simulink model "tp320031"  (Simulink 3.0)
settings: Solver=ode1  SolverMode=SingleTasking  StartTime=0.0  StopTime=t_sim  FixedStep=Ts  RelTol=1e-3
values from neighbouring files (symbols this model uses):
  t_prep = 80    [step_resp1.mat]
  Ts = 0.2    [init_I0_disc2.m]    (also in init_PI0_windupless.m = 0.5; init_PI1_windupless.m; init_PID.m; step_resp1.mat)
  Umax = 5    [init_I0_disc2.m]    (also in init_PI0_windupless.m; init_PI1_windupless.m; init_PID.m; step_resp1.mat)
  Umin = 0    [init_I0_disc2.m]    (also in init_PI0_windupless.m; init_PI1_windupless.m; init_PID.m; step_resp1.mat)
  w = 20    [step_resp1.mat]
undefined symbols (not defined in the file or in its folder): t_step
libraries: udaq28LT_lib x1
settings Model: LastModifiedBy=mato  SaveFormat=Matrix  BooleanDataType=on

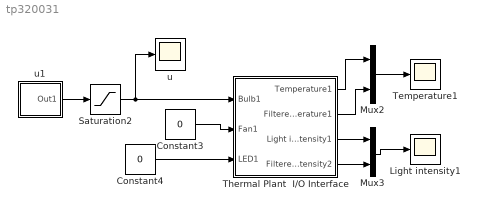
== system tp320031 ==
  Constant3 : Constant  Value=0
  Constant4 : Constant  Value=0
  Light intensity1 : Scope
      settings: TickLabels=on  TimeRange=30  YMin=0  YMax=100  SaveName=yl  DataFormat=Matrix
  Mux2 : Mux  Inputs=2
  Mux3 : Mux  Inputs=2
  Saturation2 : Saturate  UpperLimit=Umax  LowerLimit=Umin
  Temperature1 : Scope
      settings: TickLabels=on  TimeRange=30  YMin=15  YMax=50  SaveName=yt  DataFormat=Matrix
  Thermal Plant  I/O Interface : Subsystem
      mask Display: disp('Thermo-optical\nPlant\nI/O Interface')
  u : Scope
      settings: TimeRange=33  YMin=-0.5  YMax=5.5  SaveName=u  DataFormat=Matrix  Decimation=10  SampleInput=on  SampleTime=Ts
  u1 : Subsystem
  wires:
  Saturation2/1 -> u/1, Thermal Plant  I/O Interface/1(Bulb1)
  u1/1(Out1) -> Saturation2/1
  Mux3/1 -> Light intensity1/1
  Mux2/1 -> Temperature1/1
  Constant3/1 -> Thermal Plant  I/O Interface/2(Fan1)
  Constant4/1 -> Thermal Plant  I/O Interface/3(LED1)
  Thermal Plant  I/O Interface/1(Temperature1) -> Mux2/1
  Thermal Plant  I/O Interface/2(Filtered  temperature1) -> Mux2/2
  Thermal Plant  I/O Interface/3(Light intensity1) -> Mux3/1
  Thermal Plant  I/O Interface/4(Filtered  light intensity2) -> Mux3/2

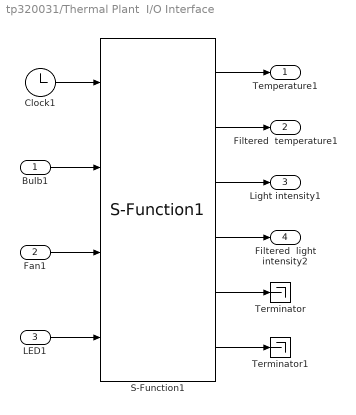
== system tp320031/Thermal Plant  I/O Interface ==
  Bulb1 : Inport  Port=1  PortWidth=-1  SampleTime=-1  DataType=auto
      settings: SignalType=auto
  Fan1 : Inport  Port=2  PortWidth=-1  SampleTime=-1  DataType=auto
      settings: SignalType=auto
  LED1 : Inport  Port=3  PortWidth=-1  SampleTime=-1  DataType=auto
      settings: SignalType=auto
  Clock1 : Clock
      settings: DisplayTime=off  Decimation=10
  S-Function1 : udaq28LT_lib/S-Function1  Priority=1  com_port=COM3  Ts=Ts  events_ot=2  rd_timeout=Ts/2*1000  matlab_prior=ABOVE_NORMAL_PRIORITY  warning=on  printout=off
  Terminator : Terminator
  Terminator1 : Terminator
  Temperature1 : Outport  Port=1
  Filtered  temperature1 : Outport  Port=2
  Light intensity1 : Outport  Port=3
  Filtered  light intensity2 : Outport  Port=4
  wires:
  S-Function1/1 -> Temperature1/1
  S-Function1/2 -> Filtered  temperature1/1
  Clock1/1 -> S-Function1/1
  Bulb1/1 -> S-Function1/2
  Fan1/1 -> S-Function1/3
  S-Function1/3 -> Light intensity1/1
  S-Function1/4 -> Filtered  light intensity2/1
  S-Function1/5 -> Terminator/1
  S-Function1/6 -> Terminator1/1
  LED1/1 -> S-Function1/4

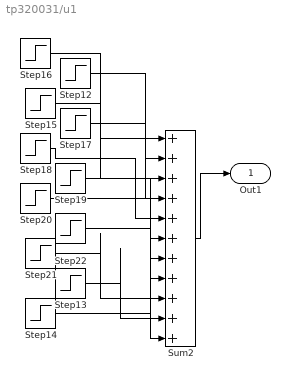
== system tp320031/u1 ==
  Step12 : Step  Time=t_prep+1*t_step  Before=0  After=w(2)-w(1)  SampleTime=Ts
  Step13 : Step  Time=t_prep+9*t_step  Before=0  After=w(2)-w(1)  SampleTime=Ts
  Step14 : Step  Time=t_prep+10*t_step  Before=0  After=w(2)-w(1)  SampleTime=Ts
  Step15 : Step  Time=t_prep+2*t_step  Before=0  After=w(2)-w(1)  SampleTime=Ts
  Step16 : Step  Time=t_prep  Before=0  After=Umin  SampleTime=Ts
  Step17 : Step  Time=t_prep+3*t_step  Before=0  After=w(2)-w(1)  SampleTime=Ts
  Step18 : Step  Time=t_prep+4*t_step  Before=0  After=w(2)-w(1)  SampleTime=Ts
  Step19 : Step  Time=t_prep+5*t_step  Before=0  After=w(2)-w(1)  SampleTime=Ts
  Step20 : Step  Time=t_prep+6*t_step  Before=0  After=w(2)-w(1)  SampleTime=Ts
  Step21 : Step  Time=t_prep+8*t_step  Before=0  After=w(2)-w(1)  SampleTime=Ts
  Step22 : Step  Time=t_prep+7*t_step  Before=0  After=w(2)-w(1)  SampleTime=Ts
  Sum2 : Sum  Inputs=|+++++++++++  SaturateOnIntegerOverflow=on
  Out1 : Outport  Port=1
  wires:
  Step14/1 -> Sum2/11
  Step16/1 -> Sum2/1
  Step12/1 -> Sum2/2
  Step15/1 -> Sum2/3
  Step17/1 -> Sum2/4
  Step18/1 -> Sum2/5
  Step19/1 -> Sum2/6
  Step20/1 -> Sum2/7
  Step22/1 -> Sum2/8
  Step21/1 -> Sum2/9
  Step13/1 -> Sum2/10
  Sum2/1 -> Out1/1
